simulink model "water_tank_control"  (R2021a)
settings: Solver=ode45  StartTime=0  StopTime=100  MaxStep=0.2  RelTol=1e-3  AbsTol=1e-6
PreLoadFcn:
  | tank=readfis('tank');
libraries: fuzblock x1, pid_lib x1
CloseFcn:
  | AnimFigH = findobj(0,'Name', 'Tank Demo'); close(AnimFigH)
  | 
  | clear tank AnimFigH
settings Model: FPTRunName=Active  Creator=The MathWorks, Inc.  LastModifiedBy=hp
settings SolverCC: AutoScaleAbsTol=off  AlgebraicLoopSolver=TrustRegion
settings DataIOCC: SaveFormat=Array  SaveOutput=off  SaveTime=off  ReturnWorkspaceOutputs=off
settings OptimizationCC: BlockReduction=off  BooleanDataType=off  ExpressionDepthLimit=2147483647  InitFltsAndDblsToZero=on  LifeSpan=inf
settings DebuggingCC: SaveWithParameterizedLinksMsg=none  UnderspecifiedInitializationDetection=Classic  MergeDetectMultiDrivingBlocksExec=none  SignalResolutionControl=TryResolveAllWithWarning  MultiTaskDSMMsg=warning  MultiTaskCondExecSysMsg=none  FcnCallInpInsideContextMsg=warning  StateNameClashWarn=warning  SFUnexpectedBacktrackingDiag=warning  SFNoUnconditionalDefaultTransitionDiag=warning  SFExecutionAtInitializationDiag=none  SFMachineParentedDataDiag=warning  ArithmeticOperatorsInVariantConditions=warning
settings HardwareCC: ProdBitPerPointer=32  ProdBitPerSizeT=32  ProdBitPerPtrDiffT=32  ProdLargestAtomicFloat=None  ProdIntDivRoundTo=Undefined  ProdEndianess=Unspecified  ProdWordSize=32  ProdHWDeviceType=32-bit Generic  TargetUnknown=on
settings ModelReferenceCC: PropagateSignalLabelsOutOfModel=off
settings SFSimCC: SimUseLocalCustomCode=off  CustomCodeUndefinedFunction=UseInterfaceOnly
settings RTWCC: TemplateMakefile=grt_unix.tmf  RTWUseLocalCustomCode=off
settings CodeAppCC: StateflowObjectComments=on
settings GRTTargetCC: TargetFcnLib=ansi_tfl_tmw.mat  TargetLangStandard=C89/C90 (ANSI)  CombineOutputUpdateFcns=off  GRTInterface=on
settings ConfigComp: CovMetricSettings=dw  CovSaveCumulativeToWorkspaceVar=on  CovSaveSingleToWorkspaceVar=on  CovExternalEMLEnable=off

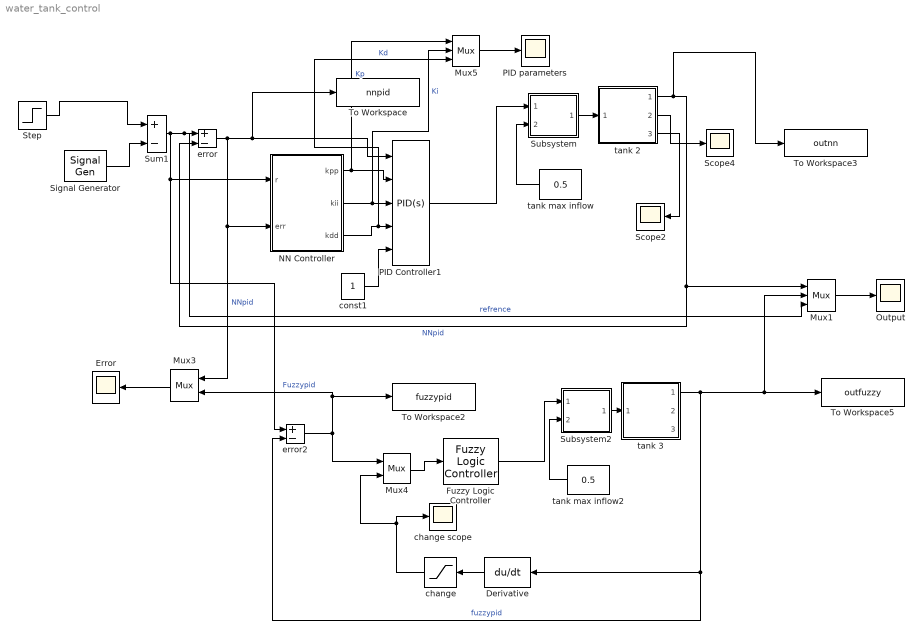
== system water_tank_control ==
  Derivative : Derivative
  Error : Scope
  Fuzzy Logic Controller : fuzblock/Fuzzy Logic  Controller  FIS=tank  OutputSampleNumber=101  DataType=double  FuzzifiedInputs=off  RuleFiringStrengths=off  RuleOutputs=off  AggregatedOutputs=off  SimulateUsing=Interpreted execution  OutOfRangeInputValueMessage=warning  NoRuleFiredMessage=warning  EmptyOutputFuzzySetMessage=warning
  Mux1 : Mux  Inputs=3
  Mux3 : Mux  Inputs=2
  Mux4 : Mux  Inputs=2
  Mux5 : Mux  Inputs=3
  NN Controller : MATLAB Function  TreatAsAtomicUnit=on
  Output : Scope
  PID Controller1 : pid_lib/PID Controller  Controller=PID  Form=Parallel  TimeDomain=Continuous-time  UseExternalTs=off  SampleTime=1  IntegratorMethod=Forward Euler  FilterMethod=Forward Euler  ControllerParametersSource=external  P=2  I=0  D=1  UseFilter=on  N=100  TunerSelectOption=Transfer Function Based (PID Tuner App)  InitialConditionSource=internal  InitialConditionForIntegrator=0  InitialConditionForFilter=0  DifferentiatorICPrevScaledInput=0  ExternalReset=none  TrackingMode=off  Kt=1  LimitOutput=on  SatLimitsSource=internal  UpperSaturationLimit=inf  LowerSaturationLimit=-inf  LinearizeAsGain=off  AntiWindupMode=back-calculation  Kb=1  POutMin=[]  POutMax=[]  IOutMin=[]  IOutMax=[]  DOutMin=[]  DOutMax=[]  NOutMin=[]  NOutMax=[]  SumOutMin=[]  SumOutMax=[]  SaturationOutMin=[]  SaturationOutMax=[]  PParamMin=[]  PParamMax=[]  IParamMin=[]  IParamMax=[]  DParamMin=[]  DParamMax=[]  NParamMin=[]  NParamMax=[]  KbParamMin=[]  KbParamMax=[]  KtParamMin=[]  KtParamMax=[]  KbOutMin=[]  KbOutMax=[]  KtOutMin=[]  KtOutMax=[]  IntegratorOutMin=[]  IntegratorOutMax=[]  FilterOutMin=[]  FilterOutMax=[]  SumI1OutMin=[]  SumI1OutMax=[]  SumI2OutMin=[]  SumI2OutMax=[]  SumI3OutMin=[]  SumI3OutMax=[]  SumI4OutMin=[]  SumI4OutMax=[]  SumDOutMin=[]  SumDOutMax=[]  DifferentiatorOutMin=[]  DifferentiatorOutMax=[]  FilterDiffOutCoefMin=[]  FilterDiffOutCoefMax=[]  ReciprocalOutMin=[]  ReciprocalOutMax=[]  SumDenOutMin=[]  SumDenOutMax=[]  SumNumOutMin=[]  SumNumOutMax=[]  DivideOutMin=[]  DivideOutMax=[]  UdiffTsProdOutMin=[]  UdiffTsProdOutMax=[]  NTsProdOutMin=[]  NTsProdOutMax=[]  UintegralTsProdOutMin=[]  UintegralTsProdOutMax=[]  UngainTsProdOutMin=[]  UngainTsProdOutMax=[]  IntegratorContinuousStateAttributes=''  IntegratorStateMustResolveToSignalObject=off  IntegratorRTWStateStorageClass=Auto  FilterContinuousStateAttributes=''  FilterStateMustResolveToSignalObject=off  FilterRTWStateStorageClass=Auto  ParallelPVariant=ExternalParameters  IdealPVariant=Disabled  IVariant=ExternalParameters  DVariant=ExternalParameters  IntegratorVariant=Continuous  SatVariant=Enabled  AWVariant=BackCalculation  PCopyVariant=Disabled  TRVariant=Disabled  FdbkBlocksVariant=Forward  IdealPFdbkVariant=Disabled  SatFdbkVariant=Disabled  DerivativeFilterVariant=ContFilter  NVariant=ExternalParameters  NCopyVariant=Disabled  FilterICVariant=InternalICsFilter  IntegratorICVariant=InternalICs  ExternalResetVariant=Disabled  TRSumVariant=Passthrough  SumFdbkVariant=Disabled  SumVariant=Sum_PID  TsampFilterVariant=InternalTs  TsampNgainVariant=Passthrough  TsampIntegralVariant=Passthrough  ExternalSaturationOutDataTypeStr=Inherit: Same as second input
  PID parameters : Scope
  Scope2 : Scope
  Scope4 : Scope
  Signal Generator : SignalGenerator  WaveForm=square  Amplitude=0.500000  Frequency=0.100000  Units=rad/sec
  Step : Step  Before=1  SampleTime=0
  Subsystem : Subsystem  mask(Valve){InitialPosition=0}
      mask prompts: InitialPosition "Initial position [0=closed 1=open]:"
      mask help: Valve
      mask Display: disp('VALVE')
  Subsystem2 : Subsystem  mask(Valve){InitialPosition=0}
      mask prompts: InitialPosition "Initial position [0=closed 1=open]:"
      mask help: Valve
      mask Display: disp('VALVE')
  Sum1 : Sum  Inputs=+-  InputSameDT=on  SaturateOnIntegerOverflow=on  OutDataTypeStr=Inherit: Same as first input
  To Workspace : ToWorkspace  VariableName=nnpid  SaveFormat=Timeseries  SampleTime=-1
  To Workspace2 : ToWorkspace  VariableName=fuzzypid  SaveFormat=Timeseries  SampleTime=-1
  To Workspace3 : ToWorkspace  VariableName=outnn  SaveFormat=Timeseries  SampleTime=-1
  To Workspace5 : ToWorkspace  VariableName=outfuzzy  SaveFormat=Timeseries  SampleTime=-1
  change : Saturate  UpperLimit=0.1  LowerLimit=-0.1
  change scope : Scope
  const1 : Constant
  error : Sum  Inputs=+-  InputSameDT=on  SaturateOnIntegerOverflow=on  OutDataTypeStr=Inherit: Same as first input
  error2 : Sum  Inputs=+-  InputSameDT=on  SaturateOnIntegerOverflow=on  OutDataTypeStr=Inherit: Same as first input
  tank 2 : Subsystem  mask(Water tank){ht=2, area=1, outletArea=0.05, overflowLimit=0, initialHt=0}
      mask prompts: ht "Height of tank (m):"; area "Bottom area (m^2):"; outletArea "Out pipe crossection (m^2):"; overflowLimit "Overflow sensor distance from top (m):"; initialHt "Initial level height (m):"
      mask help: Cylindrical water tank with overflow signal
      mask Display: disp('WATER\nTANK')
  tank 3 : Subsystem  mask(Water tank){ht=2, area=1, outletArea=0.05, overflowLimit=0, initialHt=0}
      mask prompts: ht "Height of tank (m):"; area "Bottom area (m^2):"; outletArea "Out pipe crossection (m^2):"; overflowLimit "Overflow sensor distance from top (m):"; initialHt "Initial level height (m):"
      mask help: Cylindrical water tank with overflow signal
      mask Display: disp('WATER\nTANK')
  tank max inflow : Constant  Value=0.5
  tank max inflow2 : Constant  Value=0.5
  wires:
  tank 2/2(flow out) -> Scope4/1
  tank max inflow/1 -> Subsystem/2(source flow)
  Signal Generator/1 -> Sum1/2
  Subsystem/1(out flow) -> tank 2/1(flow in)
  tank 2/1(water level) -> To Workspace3/1, Mux1/1, error/2  "NNpid"
  Sum1/1 -> error2/1, NN Controller/1(r), Mux1/3, error/1  "refrence"
  tank 2/3(overflow flag) -> Scope2/1
  NN Controller/2(kii) -> Mux5/2, PID Controller1/3  "Ki"
  NN Controller/3(kdd) -> Mux5/3, PID Controller1/4  "Kd"
  NN Controller/1(kpp) -> PID Controller1/2, Mux5/1  "Kp"
  const1/1 -> PID Controller1/5
  Mux1/1 -> Output/1
  Mux3/1 -> Error/1
  Derivative/1 -> change/1
  tank max inflow2/1 -> Subsystem2/2(source flow)
  Mux4/1 -> Fuzzy Logic Controller/1
  Subsystem2/1(out flow) -> tank 3/1(flow in)
  tank 3/1(water level) -> error2/2, Derivative/1, Mux1/2, To Workspace5/1  "fuzzypid"
  change/1 -> Mux4/2, change scope/1
  error2/1 -> To Workspace2/1, Mux3/2, Mux4/1  "Fuzzypid"
  error/1 -> PID Controller1/1, To Workspace/1, NN Controller/2(err), Mux3/1  "NNpid"
  Mux5/1 -> PID parameters/1
  PID Controller1/1 -> Subsystem/1(control)
  Fuzzy Logic Controller/1 -> Subsystem2/1(control)
  Step/1 -> Sum1/1

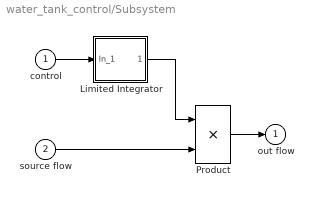
== system water_tank_control/Subsystem ==
  control : Inport
  source flow : Inport  Port=2
  Limited Integrator : Subsystem  mask(Limited integrator.){lb=0, ub=1, xi=InitialPosition}
      mask prompts: lb "Lower bound:"; ub "Upper bound:"; xi "Initial condition"
      mask help: Limited integrator
      mask Help: Implements a limited integrator with \nan expression of the form:\n\nif(x<=lb and u<0) or (x>=ub and u>0)\n\txdot=0\nelse\n\txdot=u.
      mask Display: plot(-1,-0.2,3.5,1.2,[0.05,1,2,2.9],[0,0,1,1]);disp(' 1/s    ')
  Product : Product  InputSameDT=on  RndMeth=Zero  SaturateOnIntegerOverflow=on  OutDataTypeStr=Inherit: Same as first input
  out flow : Outport  InitialOutput=0  VectorParamsAs1DForOutWhenUnconnected=off
  wires:
  source flow/1 -> Product/2
  Product/1 -> out flow/1
  control/1 -> Limited Integrator/1(In_1)
  Limited Integrator/1(Out_1) -> Product/1

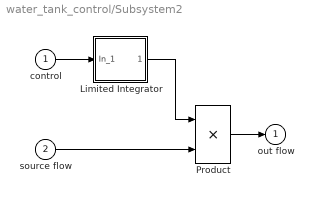
== system water_tank_control/Subsystem2 ==
  control : Inport
  source flow : Inport  Port=2
  Limited Integrator : Subsystem  mask(Limited integrator.){lb=0, ub=1, xi=InitialPosition}
      mask prompts: lb "Lower bound:"; ub "Upper bound:"; xi "Initial condition"
      mask help: Limited integrator
      mask Help: Implements a limited integrator with \nan expression of the form:\n\nif(x<=lb and u<0) or (x>=ub and u>0)\n\txdot=0\nelse\n\txdot=u.
      mask Display: plot(-1,-0.2,3.5,1.2,[0.05,1,2,2.9],[0,0,1,1]);disp(' 1/s    ')
  Product : Product  InputSameDT=on  RndMeth=Zero  SaturateOnIntegerOverflow=on  OutDataTypeStr=Inherit: Same as first input
  out flow : Outport  InitialOutput=0  VectorParamsAs1DForOutWhenUnconnected=off
  wires:
  source flow/1 -> Product/2
  Product/1 -> out flow/1
  control/1 -> Limited Integrator/1(In_1)
  Limited Integrator/1(Out_1) -> Product/1

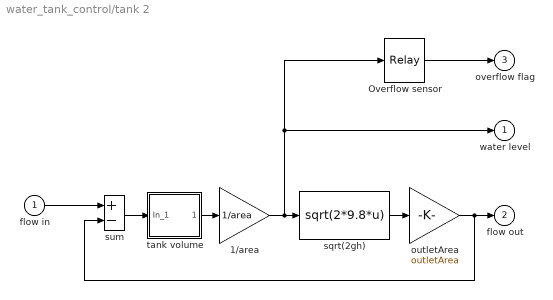
== system water_tank_control/tank 2 ==
  flow in : Inport
  1/area : Gain  Gain=1/area  SaturateOnIntegerOverflow=on  OutDataTypeStr=Inherit: Same as input  ParamDataTypeStr=Inherit: Same as input
  Overflow sensor : Relay  OnSwitchValue=ht - overflowLimit  OffSwitchValue=ht - overflowLimit
  outletArea : Gain  Gain=outletArea  SaturateOnIntegerOverflow=on  OutDataTypeStr=Inherit: Same as input  ParamDataTypeStr=Inherit: Same as input
  sqrt(2gh) : Fcn  Expr=sqrt(2*9.8*u)
  sum : Sum  Inputs=+-  InputSameDT=on  SaturateOnIntegerOverflow=on  OutDataTypeStr=Inherit: Same as first input
  tank volume : Subsystem  mask(Limited integrator.){lb=0, ub=ht * area, xi=initialHt * area}
      mask prompts: lb "Lower bound:"; ub "Upper bound:"; xi "Initial condition"
      mask help: Limited integrator
      mask Help: Implements a limited integrator with \nan expression of the form:\n\nif(x<=lb and u<0) or (x>=ub and u>0)\n\txdot=0\nelse\n\txdot=u.
      mask Display: plot(-1,-0.2,3.5,1.2,[0.05,1,2,2.9],[0,0,1,1]);disp(' 1/s    ')
  water level : Outport  InitialOutput=0  VectorParamsAs1DForOutWhenUnconnected=off
  flow out : Outport  Port=2  InitialOutput=0  VectorParamsAs1DForOutWhenUnconnected=off
  overflow flag : Outport  Port=3  InitialOutput=0  VectorParamsAs1DForOutWhenUnconnected=off
  wires:
  outletArea/1 -> flow out/1, sum/2
  sqrt(2gh)/1 -> outletArea/1
  1/area/1 -> Overflow sensor/1, water level/1, sqrt(2gh)/1
  tank volume/1(Out_1) -> 1/area/1
  Overflow sensor/1 -> overflow flag/1
  flow in/1 -> sum/1
  sum/1 -> tank volume/1(In_1)

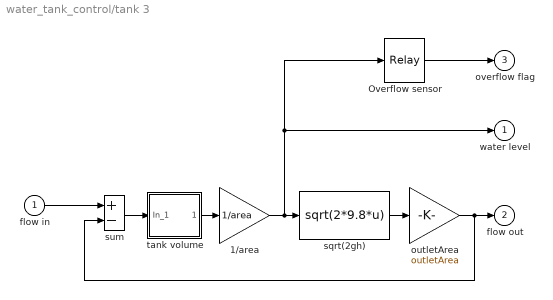
== system water_tank_control/tank 3 ==
  flow in : Inport
  1/area : Gain  Gain=1/area  SaturateOnIntegerOverflow=on  OutDataTypeStr=Inherit: Same as input  ParamDataTypeStr=Inherit: Same as input
  Overflow sensor : Relay  OnSwitchValue=ht - overflowLimit  OffSwitchValue=ht - overflowLimit
  outletArea : Gain  Gain=outletArea  SaturateOnIntegerOverflow=on  OutDataTypeStr=Inherit: Same as input  ParamDataTypeStr=Inherit: Same as input
  sqrt(2gh) : Fcn  Expr=sqrt(2*9.8*u)
  sum : Sum  Inputs=+-  InputSameDT=on  SaturateOnIntegerOverflow=on  OutDataTypeStr=Inherit: Same as first input
  tank volume : Subsystem  mask(Limited integrator.){lb=0, ub=ht * area, xi=initialHt * area}
      mask prompts: lb "Lower bound:"; ub "Upper bound:"; xi "Initial condition"
      mask help: Limited integrator
      mask Help: Implements a limited integrator with \nan expression of the form:\n\nif(x<=lb and u<0) or (x>=ub and u>0)\n\txdot=0\nelse\n\txdot=u.
      mask Display: plot(-1,-0.2,3.5,1.2,[0.05,1,2,2.9],[0,0,1,1]);disp(' 1/s    ')
  water level : Outport  InitialOutput=0  VectorParamsAs1DForOutWhenUnconnected=off
  flow out : Outport  Port=2  InitialOutput=0  VectorParamsAs1DForOutWhenUnconnected=off
  overflow flag : Outport  Port=3  InitialOutput=0  VectorParamsAs1DForOutWhenUnconnected=off
  wires:
  outletArea/1 -> flow out/1, sum/2
  sqrt(2gh)/1 -> outletArea/1
  1/area/1 -> Overflow sensor/1, water level/1, sqrt(2gh)/1
  tank volume/1(Out_1) -> 1/area/1
  Overflow sensor/1 -> overflow flag/1
  flow in/1 -> sum/1
  sum/1 -> tank volume/1(In_1)

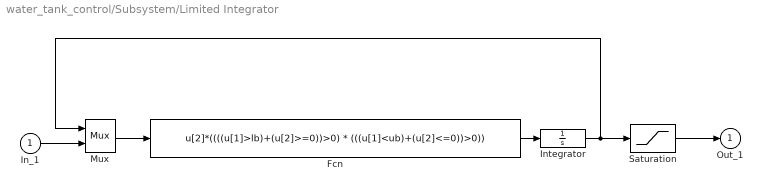
== system water_tank_control/Subsystem/Limited Integrator ==
  In_1 : Inport
  Fcn : Fcn  Expr=u[2]*((((u[1]>lb)+(u[2]>=0))>0) * (((u[1]<ub)+(u[2]<=0))>0))
  Integrator : Integrator  InitialCondition=xi
  Mux : Mux  Inputs=2
  Saturation : Saturate  UpperLimit=ub  LowerLimit=lb
  Out_1 : Outport  InitialOutput=0  VectorParamsAs1DForOutWhenUnconnected=off
  wires:
  Integrator/1 -> Saturation/1, Mux/1
  Fcn/1 -> Integrator/1
  Mux/1 -> Fcn/1
  In_1/1 -> Mux/2
  Saturation/1 -> Out_1/1

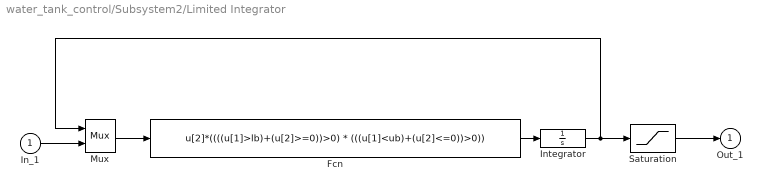
== system water_tank_control/Subsystem2/Limited Integrator ==
  In_1 : Inport
  Fcn : Fcn  Expr=u[2]*((((u[1]>lb)+(u[2]>=0))>0) * (((u[1]<ub)+(u[2]<=0))>0))
  Integrator : Integrator  InitialCondition=xi
  Mux : Mux  Inputs=2
  Saturation : Saturate  UpperLimit=ub  LowerLimit=lb
  Out_1 : Outport  InitialOutput=0  VectorParamsAs1DForOutWhenUnconnected=off
  wires:
  Integrator/1 -> Saturation/1, Mux/1
  Fcn/1 -> Integrator/1
  Mux/1 -> Fcn/1
  In_1/1 -> Mux/2
  Saturation/1 -> Out_1/1

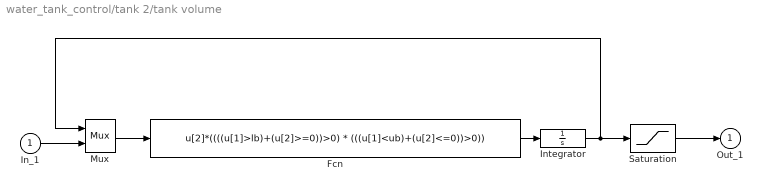
== system water_tank_control/tank 2/tank volume ==
  In_1 : Inport
  Fcn : Fcn  Expr=u[2]*((((u[1]>lb)+(u[2]>=0))>0) * (((u[1]<ub)+(u[2]<=0))>0))
  Integrator : Integrator  InitialCondition=xi
  Mux : Mux  Inputs=2
  Saturation : Saturate  UpperLimit=ub  LowerLimit=lb
  Out_1 : Outport  InitialOutput=0  VectorParamsAs1DForOutWhenUnconnected=off
  wires:
  Integrator/1 -> Saturation/1, Mux/1
  Fcn/1 -> Integrator/1
  Mux/1 -> Fcn/1
  In_1/1 -> Mux/2
  Saturation/1 -> Out_1/1

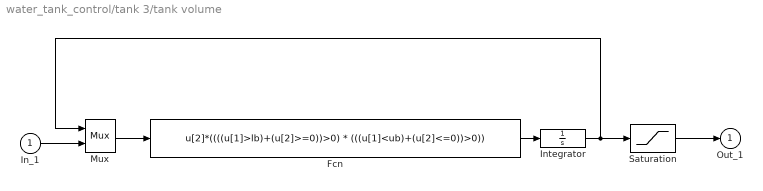
== system water_tank_control/tank 3/tank volume ==
  In_1 : Inport
  Fcn : Fcn  Expr=u[2]*((((u[1]>lb)+(u[2]>=0))>0) * (((u[1]<ub)+(u[2]<=0))>0))
  Integrator : Integrator  InitialCondition=xi
  Mux : Mux  Inputs=2
  Saturation : Saturate  UpperLimit=ub  LowerLimit=lb
  Out_1 : Outport  InitialOutput=0  VectorParamsAs1DForOutWhenUnconnected=off
  wires:
  Integrator/1 -> Saturation/1, Mux/1
  Fcn/1 -> Integrator/1
  Mux/1 -> Fcn/1
  In_1/1 -> Mux/2
  Saturation/1 -> Out_1/1

== matlab function water_tank_control/NN Controller ==
  settings: updateMethod=DISCRETE  sampleTime=1
  data: r input; err input; kpp output; kii output; kdd output
function [kpp, kii, kdd]  = fcn(r,err)
persistent Wij_c_p W1j_c_p S_prev_c_p e_prev_c_p u_prev_c_p u_prev_e_P control_prev
        if isempty(Wij_c_p)
        Wij_c_p = 0.05*rand(4,4);
        end
        if isempty(W1j_c_p)
        W1j_c_p = 0.05*rand(1,4);
        end
        if isempty(S_prev_c_p)
        S_prev_c_p = [0.1 0.2 0.3 0.4];
        end
        if isempty(e_prev_c_p)
        e_prev_c_p = 1;
        end
        if isempty(err)
        err = 1;
        end
        if isempty(u_prev_c_p)
        u_prev_c_p = 0;
        end
        if isempty(u_prev_e_P)
        u_prev_e_P = 0.05;
        end
        if isempty(control_prev)
        control_prev = 0;
        end
       % ********
           persistent e e_prev1 e_prev2 e_prev3 error_status
       error_status = 1;
       while true
            if isempty(e)
                e = err
                e_prev1 = 1
                e_prev2 = 1
                e_prev3 = 1
                error_status = 2;
                break
            elseif error_status == 2
                e_prev1 = e
                e = err
                e_prev2
                e_prev3
                error_status = 3
                break
            elseif error_status == 3
                e_prev2 = e_prev1
                e_prev1  = e
                e = err
                e_prev3
                error_status == 4
                break
            elseif error_status == 4
                e_prev3 =e_prev2
                e_prev2 = e_prev1
                e_prev1 = e
                e = err
                error_status == 5
                break
            else
                e_prev3 =e_prev2
                e_prev2 = e_prev1
                e_prev1 = e
                e = err
                break
            end
       end
       %***********
       persistent xp xp_prev1 xp_prev2 xp_prev3 xp_status
       xp_status = 1;
       while true
            if isempty(xp)
                xp = r
                xp_prev1 = 1
                xp_prev2 = 1
                xp_prev3 = 1
                xp_status = 2;
                break
            elseif xp_status == 2
                xp_prev1 = xp
                xp = r
                xp_prev2
                xp_prev3
                xp_status = 3
                break
            elseif xp_status == 3
                xp_prev2 = xp_prev1
                xp_prev1  = xp
                xp = r
                xp_prev3
                xp_status == 4
                break
            elseif xp_status == 4
                xp_prev3 =xp_prev2
                xp_prev2 = xp_prev1
                xp_prev1 = xp
                xp = r
                xp_status == 5
                break
            else
                xp_prev3 =xp_prev2
                xp_prev2 = xp_prev1
                xp_prev1 = xp
                xp = r
                break
            end
       end
       %******
       persistent Kp Ki Kd Kp_prev Ki_prev Kd_prev
        if isempty(Kp)
        Kp = 200;
        end
        if isempty(Ki)
        Ki = 3.5;
        end
        if isempty(Kd)
        Kd = 0.0043;
        end
        if isempty(Kp_prev)
        Kp_prev = 0;
        end
        if isempty(Ki_prev)
        Ki_prev = 0;
        end
        if isempty(Kd_prev)
        Kd_prev = 0;
        end

% input layer
net1_c_p = [xp;xp_prev1;xp_prev2;xp_prev3];
O1_c_p = net1_c_p;

% hidden layyer 
S_c_p = zeros (1,4);
 for j = 1:4
       S_c_p(j) = tanh(Wij_c_p(j,1)*xp+Wij_c_p(j,2)*xp_prev1 + Wij_c_p(j,3)*xp_prev2 + Wij_c_p(j,4)*xp_prev3);
 end
O2_c_p = zeros(1,4);
O2_c_p = [S_c_p(1),S_c_p(2),S_c_p(3),S_c_p(4)];

%output layer
net3_c_p = 0;
net3_c_p = W1j_c_p.*O2_c_p;
u_c_p = 0.5*(1+tanh(net3_c_p(1,1)+ net3_c_p(1,2) + net3_c_p(1,3)+net3_c_p(1,4)));

%% updating weights
B_c_p = 0.025;
d_c_p = u_prev_e_P;
sigma_c_p = sqrt(B_c_p)*e_prev1 + d_c_p;

%W1j updating
for j = 1 :4
    W1j_c_p(j) = sigma_c_p/(4*(S_prev_c_p(j))); %changed it to mean spc
end

%Wij updating
for j = 1:4
    Wij_c_p(j,1) = (1/(4*xp))*atanh(sigma_c_p/(4*W1j_c_p(1,j))); % Not OK
end
for j = 1:4
    Wij_c_p(j,2) = (1/(4*xp_prev1))*atanh(sigma_c_p/(4*W1j_c_p(1,j))); % Not OK
end
for j = 1:4
    Wij_c_p(j,3) = (1/(4*xp_prev2))*atanh(sigma_c_p/(4*W1j_c_p(1,j))); % Not OK
end
for j = 1:4
    Wij_c_p(j,4) = (1/(4*xp_prev3))*atanh(sigma_c_p/(4*W1j_c_p(1,j))); % Not OK
end

%% NNE
persistent Wij_e_p W1j_e_p S_prev_e_p e_prev_e_p  
        if isempty(Wij_e_p)
        Wij_e_p = 0.05*rand(4,4);
        end
        if isempty(W1j_e_p)
        W1j_e_p = 0.05*rand(1,4);
        end
        if isempty(S_prev_e_p)
        S_prev_e_p = [0.1 0.2 0.3 0.4];
        end
        if isempty(e_prev_e_p)
        e_prev_e_p = 1;
        end
    
% input layer
net1_e_p = [xp;xp_prev1;xp_prev2;xp_prev3];
O1_e_p = net1_e_p;

% hidden layyer 
S_e_p = zeros (1,4);
 for j = 1:4
       S_e_p(j) = tanh(Wij_e_p(j,1)*xp+Wij_e_p(j,2)*xp_prev1 + Wij_e_p(j,3)*xp_prev2 + Wij_e_p(j,4)*xp_prev3);
 end
O2_e_p = zeros(1,4);
O2_e_p = [S_e_p(1),S_e_p(2),S_e_p(3),S_e_p(4)];

%output layer
net3_e_p = 0;
net3_e_p = W1j_e_p.*O2_e_p;
u_e_p = 0.5*(1+tanh(net3_e_p(1,1)+ net3_e_p(1,2) + net3_e_p(1,3)+net3_e_p(1,4)));

%% updating weights
e_e_p = u_e_p - u_c_p;
B_e_p = 0.025;
d_e_p = u_c_p;
sigma_e_p = sqrt(B_e_p)*e_prev_e_p + d_e_p;
for j = 1 :4
    W1j_e_p(j) = sigma_e_p/(4*(S_prev_e_p(j))); %changed it to mean spc
end

for j = 1:4
    Wij_e_p(j,1) = (1/(4*xp))*atanh(sigma_e_p/(4*W1j_e_p(1,j))); % Not OK
end
for j = 1:4
    Wij_e_p(j,2) = (1/(4*xp_prev1))*atanh(sigma_e_p/(4*W1j_e_p(1,j))); % Not OK
end
for j = 1:4
    Wij_e_p(j,3) = (1/(4*xp_prev2))*atanh(sigma_e_p/(4*W1j_e_p(1,j))); % Not OK
end
for j = 1:4
    Wij_e_p(j,4) = (1/(4*xp_prev3))*atanh(sigma_e_p/(4*W1j_e_p(1,j))); % Not OK
end
u_c_p = u_c_p*800;
%**************
S_prev_c_p = S_c_p;
e_prev_c_p = err;
S_prev_e_p = S_e_p;
e_prev_e_p = e_e_p;
u_prev_e_P = u_e_p;

%% NNI
persistent Wij_c_i W1j_c_i S_prev_c_i e_prev_c_i u_prev_c_i u_prev_e_i error_integral
    if isempty(Wij_c_i)
        Wij_c_i = 0.05*rand(4,4);
    end
    if isempty(W1j_c_i)
        W1j_c_i = 0.05*rand(1,4);
    end
        if isempty(S_prev_c_i)
        S_prev_c_i = [0.1 0.2 0.3 0.4];
        end
        if isempty(e_prev_c_i)
        e_prev_c_i = 1;
        end
        if isempty(err)
        err = 1;
        end
        if isempty(u_prev_c_i)
        u_prev_c_i = 0;
        end
        if isempty(u_prev_e_i)
        u_prev_e_i = 0.05;
        end
        if isempty(error_integral)
        error_integral = 1;
        end

    
% input layer
net1_c_i = [xp;xp_prev1;xp_prev2;xp_prev3];
O1_c_i = net1_c_i;

% hidden layyer 
S_c_i = zeros (1,4);
 for j = 1:4
       S_c_i(j) = tanh(Wij_c_i(j,1)*xp+Wij_c_i(j,2)*xp_prev1 + Wij_c_i(j,3)*xp_prev2 + Wij_c_i(j,4)*xp_prev3);
 end
O2_c_i = zeros(1,4);
O2_c_i = [S_c_i(1),S_c_i(2),S_c_i(3),S_c_i(4)]; 
%output layer
net3_c_i = 0;
net3_c_i = W1j_c_i.*O2_c_i;
u_c_i = 0.5*(1+tanh(net3_c_i(1,1)+ net3_c_i(1,2) + net3_c_i(1,3)+net3_c_i(1,4)));

%% updating weights
B_c_i = 0.025;
d_c_i = u_prev_e_i;
sigma_c_i = sqrt(B_c_i)*error_integral + d_c_i;
error_integral = e + error_integral;
for j = 1 :4
    W1j_c_i(j) = sigma_c_i/(4*(S_prev_c_i(j))); %changed it to mean spc
end

for j = 1:4
    Wij_c_i(j,1) = (1/(4*xp))*atanh(sigma_c_i/(4*W1j_c_i(1,j))); % Not OK
end
for j = 1:4
    Wij_c_i(j,2) = (1/(4*xp_prev1))*atanh(sigma_c_i/(4*W1j_c_i(1,j))); % Not OK
end
for j = 1:4
    Wij_c_i(j,3) = (1/(4*xp_prev2))*atanh(sigma_c_i/(4*W1j_c_i(1,j))); % Not OK
end
for j = 1:4
    Wij_c_i(j,4) = (1/(4*xp_prev3))*atanh(sigma_c_i/(4*W1j_c_i(1,j))); % Not OK
end

%% NNE
persistent Wij_e_i W1j_e_i S_prev_e_i e_prev_e_i  
    if isempty(Wij_e_i)
        Wij_e_i = 0.05*rand(4,4);
    end
    if isempty(W1j_e_i)
        W1j_e_i = 0.05*rand(1,4);
    end
        if isempty(S_prev_e_i)
        S_prev_e_i = [0.1 0.2 0.3 0.4];
        end
        if isempty(e_prev_e_i)
        e_prev_e_i = 1;
        end
    
% input layer
net1_e_i = [xp;xp_prev1;xp_prev2;xp_prev3];
O1_e_i = net1_e_i;
% hidden layyer 
S_e_i = zeros (1,4);
 for j = 1:4
       S_e_i(j) = tanh(Wij_e_i(j,1)*xp+Wij_e_i(j,2)*xp_prev1 + Wij_e_i(j,3)*xp_prev2 + Wij_e_i(j,4)*xp_prev3);
 end
O2_e_i = zeros(1,4);
O2_e_i = [S_e_i(1),S_e_i(2),S_e_i(3),S_e_i(4)]; 
%output layer
net3_e_i = 0;
net3_e_i = W1j_e_i.*O2_e_i;
u_e_i = 0.5*(1+tanh(net3_e_i(1,1)+ net3_e_i(1,2) + net3_e_i(1,3)+net3_e_i(1,4)));

%% updating weights
e_e_i = u_e_i - u_c_i;
B_e_i = 0.025;
d_e_i = u_c_i;
sigma_e_i = sqrt(B_e_i)*e_prev_e_i + d_e_i;
for j = 1 :4
    W1j_e_i(j) = sigma_e_i/(4*(S_prev_e_i(j))); %changed it to mean spc
end

for j = 1:4
    Wij_e_i(j,1) = (1/(4*xp))*atanh(sigma_e_i/(4*W1j_e_i(1,j))); % Not OK
end
for j = 1:4
    Wij_e_i(j,2) = (1/(4*xp_prev1))*atanh(sigma_e_i/(4*W1j_e_i(1,j))); % Not OK
end
for j = 1:4
    Wij_e_i(j,3) = (1/(4*xp_prev2))*atanh(sigma_e_i/(4*W1j_e_i(1,j))); % Not OK
end
for j = 1:4
    Wij_e_i(j,4) = (1/(4*xp_prev3))*atanh(sigma_e_i/(4*W1j_e_i(1,j))); % Not OK
end
u_c_i = u_c_i*0.1;
%**************
S_prev_c_i = S_c_i;
e_prev_c_i = err;
S_prev_e_i = S_e_i;
e_prev_e_i = e_e_i;
u_prev_e_i = u_e_i;

%% NND
persistent Wij_c_d W1j_c_d S_prev_c_d e_prev_c_d u_prev_c_d u_prev_e_d error_derivative
    if isempty(Wij_c_d)
        Wij_c_d = 0.05*rand(4,4);
    end
    if isempty(W1j_c_d)
        W1j_c_d = 0.05*rand(1,4);
    end
        if isempty(S_prev_c_d)
        S_prev_c_d = [0.1 0.2 0.3 0.4];
        end
        if isempty(e_prev_c_d)
        e_prev_c_d = 1;
        end
        if isempty(u_prev_c_d)
        u_prev_c_d = 0;
        end
        if isempty(u_prev_e_d)
        u_prev_e_d = 0.05;
        end
        if isempty(error_derivative)
        error_derivative = 1;
        end

   
% input layer
net1_c_d = [xp;xp_prev1;xp_prev2;xp_prev3];
O1_c_d = net1_c_d;
% hidden layyer 
S_c_d = zeros (1,4);
 for j = 1:4
       S_c_d(j) = tanh(Wij_c_d(j,1)*xp+Wij_c_d(j,2)*xp_prev1 + Wij_c_d(j,3)*xp_prev2 + Wij_c_d(j,4)*xp_prev3);
 end

O2_c_d = zeros(1,4);
O2_c_d = [S_c_d(1),S_c_d(2),S_c_d(3),S_c_d(4)]; 
%output layer
net3_c_d = 0;
net3_c_d = W1j_c_d.*O2_c_d;
u_c_d = 0.5*(1+tanh(net3_c_d(1,1)+ net3_c_d(1,2) + net3_c_d(1,3)+net3_c_d(1,4)));

%% updating weights
B_c_d = 0.025;
d_c_d = u_prev_e_d;

sigma_c_d = sqrt(B_c_d)*error_derivative + d_c_d;
 error_derivative = (e - e_prev1)/0.002; %need to be fixed
for j = 1 :4
    W1j_c_d(j) = sigma_c_d/(4*(S_prev_c_d(j))); %changed it to mean spc
end
% W1j = sigma / (4*S_prev);

for j = 1:4
    Wij_c_d(j,1) = (1/(4*xp))*atanh(sigma_c_d/(4*W1j_c_d(1,j))); % Not OK
end
for j = 1:4
    Wij_c_d(j,2) = (1/(4*xp_prev1))*atanh(sigma_c_d/(4*W1j_c_d(1,j))); % Not OK
end
for j = 1:4
    Wij_c_d(j,3) = (1/(4*xp_prev2))*atanh(sigma_c_d/(4*W1j_c_d(1,j))); % Not OK
end
for j = 1:4
    Wij_c_d(j,4) = (1/(4*xp_prev3))*atanh(sigma_c_d/(4*W1j_c_d(1,j))); % Not OK
end
%% NNE
persistent Wij_e_d W1j_e_d S_prev_e_d e_prev_e_d  
    if isempty(Wij_e_d)
        Wij_e_d = 0.05*rand(4,4);
    end
    if isempty(W1j_e_d)
        W1j_e_d = 0.05*rand(1,4);
    end
        if isempty(S_prev_e_d)
        S_prev_e_d = [0.1 0.2 0.3 0.4];
        end
        if isempty(e_prev_e_d)
        e_prev_e_d = 1;
        end
    
% input layer
net1_e_d = [xp;xp_prev1;xp_prev2;xp_prev3];
O1_e_d = net1_e_d;
% hidden layyer 
S_e_d = zeros (1,4);
 for j = 1:4
       S_e_d(j) = tanh(Wij_e_d(j,1)*xp+Wij_e_d(j,2)*xp_prev1 + Wij_e_d(j,3)*xp_prev2 + Wij_e_d(j,4)*xp_prev3);
 end
O2_e_d = zeros(1,4);
O2_e_d = [S_e_d(1),S_e_d(2),S_e_d(3),S_e_d(4)]; 
%output layer
net3_e_d = 0;
net3_e_d = W1j_e_d.*O2_e_d;
u_e_d = 0.5*(1+tanh(net3_e_d(1,1)+ net3_e_d(1,2) + net3_e_d(1,3)+net3_e_d(1,4)));

%% updating weights
e_e_d = u_e_d - u_c_d;
B_e_d = 0.8;
d_e_d = u_c_d;
u_c_d= u_c_d*200;
sigma_e_d = sqrt(B_e_d)*e_prev_e_d + d_e_d;
for j = 1 :4
    W1j_e_d(j) = sigma_e_d/(4*(S_prev_e_d(j))); %changed it to mean spc
end

for j = 1:4
    Wij_e_d(j,1) = (1/(4*xp))*atanh(sigma_e_d/(4*W1j_e_d(1,j))); % Not OK
end
for j = 1:4
    Wij_e_d(j,2) = (1/(4*xp_prev1))*atanh(sigma_e_d/(4*W1j_e_d(1,j))); % Not OK
end
for j = 1:4
    Wij_e_d(j,3) = (1/(4*xp_prev2))*atanh(sigma_e_d/(4*W1j_e_d(1,j))); % Not OK
end
for j = 1:4
    Wij_e_d(j,4) = (1/(4*xp_prev3))*atanh(sigma_e_d/(4*W1j_e_d(1,j))); % Not OK
end


Kp = u_c_p;
Ki = u_c_i;
Kd = u_c_d;
Kp_prev = Kp;
Ki_prev = Ki;
Kd_prev = Kd;
kpp = Kp;
kii = Ki;
kdd = Kd;

%**************
S_prev_c_d = S_c_d;
e_prev_c_d = err;
S_prev_e_d = S_e_d;
e_prev_e_d = e_e_d;
u_prev_e_d = u_e_d;
